simulink model "spwm_inveter_lcfilter_r2023a"  (R2023a)
settings: Solver=VariableStepAuto  StartTime=0.0  StopTime=0.1  RelTol=1e-3
libraries: spsSeriesRLCBranchLib x9, spsIGBTDiodeLib x6, simulink x3, spsCurrentMeasurementLib x3, spsVoltageMeasurementLib x3, spsGroundLib x2, spsDCVoltageSourceLib x1, spsThreePhaseSeriesRLCBranchLib x1, spsTriangleGeneratorLib x1, sps_lib x1
settings Model: Creator=QUDUS  LastModifiedBy=QUDUS
settings DataIOCC: ReturnWorkspaceOutputs=off

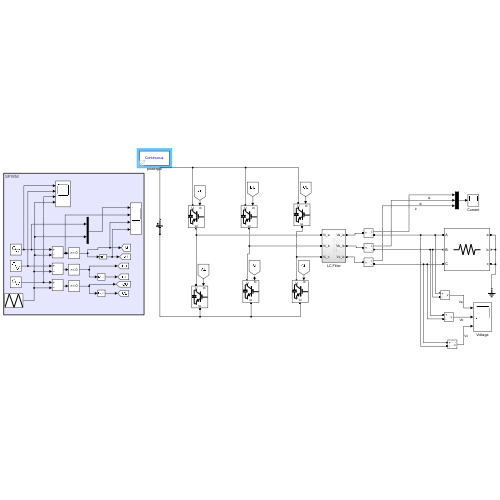
[thumbnail: Simulink's stored preview of the top-level diagram]
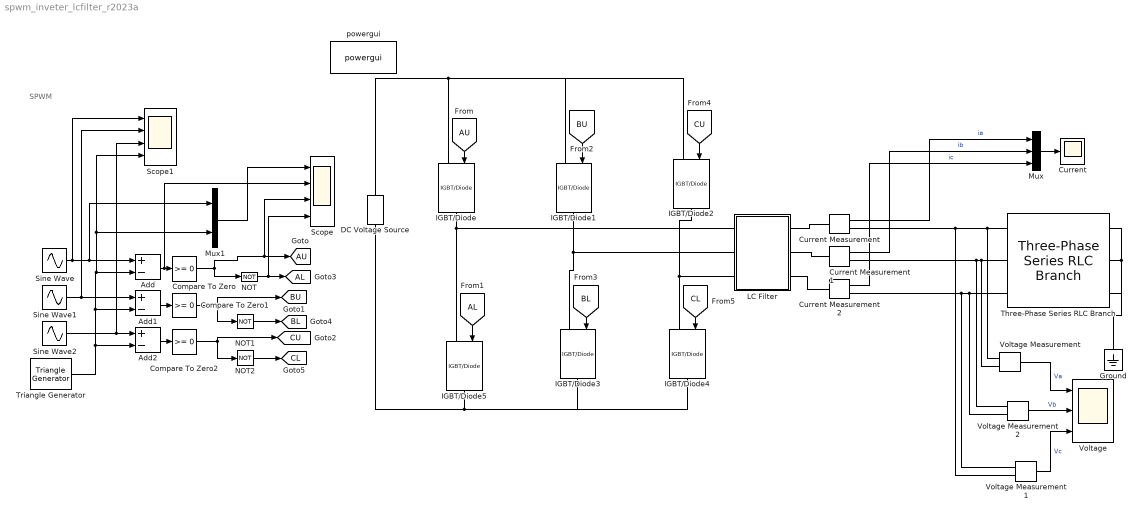
== system spwm_inveter_lcfilter_r2023a ==
  note: SPWM
  Add : Sum  Inputs=+-
  Add1 : Sum  Inputs=+-
  Add2 : Sum  Inputs=+-
  Compare To Zero : simulink/Logic and Bit Operations/Compare To Zero  relop=>=  OutDataTypeStr=boolean
  Compare To Zero1 : simulink/Logic and Bit Operations/Compare To Zero  relop=>=  OutDataTypeStr=boolean
  Compare To Zero2 : simulink/Logic and Bit Operations/Compare To Zero  relop=>=  OutDataTypeStr=boolean
  Current : Scope
  Current Measurement : spsCurrentMeasurementLib/Current Measurement  PhasorSimulation=off  OutputType=Complex  PSBequivalent=0
  Current Measurement1 : spsCurrentMeasurementLib/Current Measurement  PhasorSimulation=off  OutputType=Complex  PSBequivalent=0
  Current Measurement2 : spsCurrentMeasurementLib/Current Measurement  PhasorSimulation=off  OutputType=Complex  PSBequivalent=0
  DC Voltage Source : spsDCVoltageSourceLib/DC Voltage Source  Amplitude=440  Measurements=None
  Ground : spsGroundLib/Ground  LConnTagsString=a
  IGBT/Diode{,1..5} (6 alike) : spsIGBTDiodeLib/IGBT//Diode  Ron=1e-3  Rs=1e5  Cs=inf  Measurements=off
  LC Filter : Subsystem
  Mux : Mux  Inputs=3
  Mux1 : Mux  Inputs=2
  NOT : Logic  Operator=NOT  AllPortsSameDT=off  OutDataTypeStr=boolean
  NOT1 : Logic  Operator=NOT  AllPortsSameDT=off  OutDataTypeStr=boolean
  NOT2 : Logic  Operator=NOT  AllPortsSameDT=off  OutDataTypeStr=boolean
  Scope : Scope  NumInputPorts=4
  Scope1 : Scope  NumInputPorts=4
  Sine Wave : Sin  Frequency=2*pi*50  SampleTime=0
  Sine Wave1 : Sin  Frequency=2*pi*50  Phase=2*pi/3  SampleTime=0
  Sine Wave2 : Sin  Frequency=2*pi*50  Phase=4*pi/3  SampleTime=0
  Three-Phase Series RLC Branch : spsThreePhaseSeriesRLCBranchLib/Three-Phase Series RLC Branch  LConnTagsString=A|B|C  RConnTagsString=A|B|C  BranchType=R  Resistance=25  Inductance=1e-3  Capacitance=1e-6  Measurements=None
  Triangle Generator : spsTriangleGeneratorLib/Triangle Generator  Freq=10000  Phase=0  Ts=0
  Voltage : Scope  NumInputPorts=3
  Voltage Measurement : spsVoltageMeasurementLib/Voltage Measurement  PhasorSimulation=off  OutputType=Complex  PSBequivalent=0
  Voltage Measurement1 : spsVoltageMeasurementLib/Voltage Measurement  PhasorSimulation=off  OutputType=Complex  PSBequivalent=0
  Voltage Measurement2 : spsVoltageMeasurementLib/Voltage Measurement  PhasorSimulation=off  OutputType=Complex  PSBequivalent=0
  powergui : sps_lib/powergui  Priority=1  SimulationMode=Continuous  SampleTime=1e-6  frequency=60  Iterations=50  frequencyindice=0  Pbase=100e6  ErrMax=1e-4  UnitsV=kV  UnitsW=MW  buscounter=0  FunctionMessages=off  echomessages=off  EnableUseOfTLC=off  CurrentSourceSwitches=off  DisableSnubberDevices=off  DisableRonSwitches=off  DisableVfSwitches=off  DisplayEquations=off  AutomaticDiscreteSolvers=off  SolverType=Tustin/Backward Euler (TBE)  Interpol=off  ExternalGateDelay=off  methode=off  Ts=100  x0status=blocks  SPID=on  SwTol=0  HookPort=off  NonlinearTolerance=0  nMaxIteration=15  ContinueOnMaxIteration=off  RestoreLinks=warning  ResistiveCurrentMeasurement=off  Frange=[0:2:500]  Ylog=off  Xlog=on  ShowGrid=off  save=off  variable=ZData  structure=0  ZoomFFT=off  StartTime=0.0  cycles=1  DisplayStyle=1  fundamental=60  FreqAxis=off  MaxFrequency=1000  frequencyindicesteady=1  RmsSteady=1  display=off
  tag scope: AL=global, AU=global, BL=global, BU=global, CL=global, CU=global
  wires:
  [AU] -> IGBT/Diode/1
  [AL] -> IGBT/Diode5/1
  [CL] -> IGBT/Diode4/1
  [BL] -> IGBT/Diode3/1
  [CU] -> IGBT/Diode2/1
  [BU] -> IGBT/Diode1/1
  Mux/1 -> Current/1
  Voltage Measurement/1 -> Voltage/1  "Va"
  Voltage Measurement2/1 -> Voltage/2  "Vb"
  Voltage Measurement1/1 -> Voltage/3  "Vc"
  Mux1/1 -> Scope/1
  Compare To Zero/1 -> Scope/3, [AU], NOT/1
  Add2/1 -> Compare To Zero2/1
  NOT1/1 -> [BL]
  Add/1 -> Scope/2, Compare To Zero/1
  NOT2/1 -> [CL]
  Sine Wave1/1 -> Scope1/2, Add1/1
  NOT/1 -> Scope/4, [AL]
  Compare To Zero2/1 -> [CU], NOT2/1
  Compare To Zero1/1 -> [BU], NOT1/1
  Add1/1 -> Compare To Zero1/1
  Sine Wave/1 -> Scope1/1, Add/1, Mux1/1
  Triangle Generator/1 -> Scope1/4, Mux1/2, Add/2, Add1/2, Add2/2
  Sine Wave2/1 -> Scope1/3, Add2/1
  Current Measurement/1 -> Mux/1  "ia"
  Current Measurement1/1 -> Mux/2  "ib"
  Current Measurement2/1 -> Mux/3  "ic"
  connections:
  IGBT/Diode/LConn1 -- DC Voltage Source/RConn1 -- IGBT/Diode1/LConn1 -- IGBT/Diode2/LConn1
  Three-Phase Series RLC Branch/RConn1 -- Three-Phase Series RLC Branch/RConn3 -- Ground/LConn1 -- Three-Phase Series RLC Branch/RConn2
  DC Voltage Source/LConn1 -- IGBT/Diode4/RConn1 -- IGBT/Diode3/RConn1 -- IGBT/Diode5/RConn1
  IGBT/Diode5/LConn1 -- LC Filter/LConn1 -- IGBT/Diode/RConn1
  Three-Phase Series RLC Branch/LConn2 -- Voltage Measurement/LConn2 -- Voltage Measurement2/LConn1 -- Current Measurement1/RConn1
  Current Measurement/RConn1 -- Voltage Measurement1/LConn2 -- Voltage Measurement/LConn1 -- Three-Phase Series RLC Branch/LConn1
  Three-Phase Series RLC Branch/LConn3 -- Voltage Measurement2/LConn2 -- Voltage Measurement1/LConn1 -- Current Measurement2/RConn1
  IGBT/Diode2/RConn1 -- LC Filter/LConn3 -- IGBT/Diode4/LConn1
  IGBT/Diode1/RConn1 -- IGBT/Diode3/LConn1 -- LC Filter/LConn2
  LC Filter/RConn1 -- Current Measurement/LConn1
  LC Filter/RConn2 -- Current Measurement1/LConn1
  LC Filter/RConn3 -- Current Measurement2/LConn1

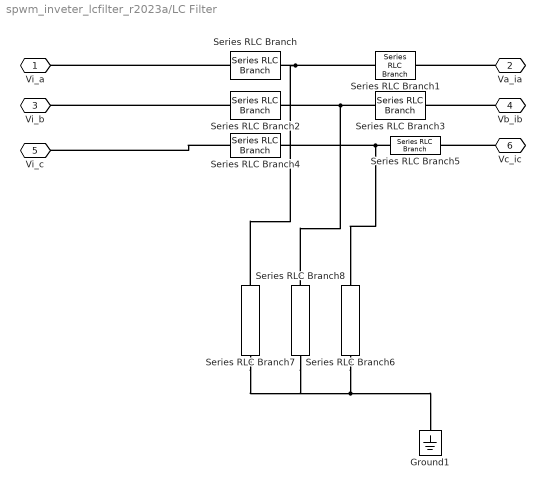
== system spwm_inveter_lcfilter_r2023a/LC Filter ==
  Ground1 : spsGroundLib/Ground  LConnTagsString=a
  Series RLC Branch{,1..5} (6 alike) : spsSeriesRLCBranchLib/Series RLC Branch  LConnTagsString=__new0  RConnTagsString=__new0  BranchType=L  Resistance=1  Inductance=1e-2  SetiL0=off  InitialCurrent=250  Capacitance=1e-6  Setx0=off  InitialVoltage=0  Measurements=None
  Series RLC Branch6 : spsSeriesRLCBranchLib/Series RLC Branch  LConnTagsString=__new0  RConnTagsString=__new0  BranchType=C  Resistance=1  Inductance=1e-3  SetiL0=off  InitialCurrent=0  Capacitance=10e-6  Setx0=off  InitialVoltage=0  Measurements=None
  Series RLC Branch7 : spsSeriesRLCBranchLib/Series RLC Branch  LConnTagsString=__new0  RConnTagsString=__new0  BranchType=C  Resistance=1  Inductance=1e-3  SetiL0=off  InitialCurrent=0  Capacitance=10e-6  Setx0=off  InitialVoltage=0  Measurements=None
  Series RLC Branch8 : spsSeriesRLCBranchLib/Series RLC Branch  LConnTagsString=__new0  RConnTagsString=__new0  BranchType=C  Resistance=1  Inductance=1e-3  SetiL0=off  InitialCurrent=0  Capacitance=10e-6  Setx0=off  InitialVoltage=0  Measurements=None
  Vi_a : PMIOPort  Side=Left
  Va_ia : PMIOPort  Port=2  Side=Right
  Vi_b : PMIOPort  Port=3  Side=Left
  Vb_ib : PMIOPort  Port=4  Side=Right
  Vi_c : PMIOPort  Port=5  Side=Left
  Vc_ic : PMIOPort  Port=6  Side=Right
  connections:
  Series RLC Branch6/RConn1 -- Series RLC Branch7/RConn1 -- Series RLC Branch8/RConn1 -- Ground1/LConn1
  Series RLC Branch1/LConn1 -- Series RLC Branch7/LConn1 -- Series RLC Branch/RConn1
  Series RLC Branch5/LConn1 -- Series RLC Branch6/LConn1 -- Series RLC Branch4/RConn1
  Va_ia/RConn1 -- Series RLC Branch1/RConn1
  Series RLC Branch3/LConn1 -- Series RLC Branch2/RConn1 -- Series RLC Branch8/LConn1
  Series RLC Branch2/LConn1 -- Vi_b/RConn1
  Vc_ic/RConn1 -- Series RLC Branch5/RConn1
  Vb_ib/RConn1 -- Series RLC Branch3/RConn1
  Series RLC Branch4/LConn1 -- Vi_c/RConn1
  Series RLC Branch/LConn1 -- Vi_a/RConn1
